simulink model "NLE_DiscreteSystem"  (R2024b)
settings: Solver=VariableStepAuto  StartTime=0.0  StopTime=20.0  RelTol=1e-3
values from neighbouring files (symbols this model uses):
  discrete_regulator = tf(Q, P, Ts)    [assignment1.m]
  disorder_times = [10, 14]    [assignment1.m]
  u_control = 0.5    [assignment1.m]
  z = 0.1    [assignment1.m]
settings Model: Creator=lukiq  LastModifiedBy=lukiq
settings DebuggingCC: AlgebraicLoopMsg=none

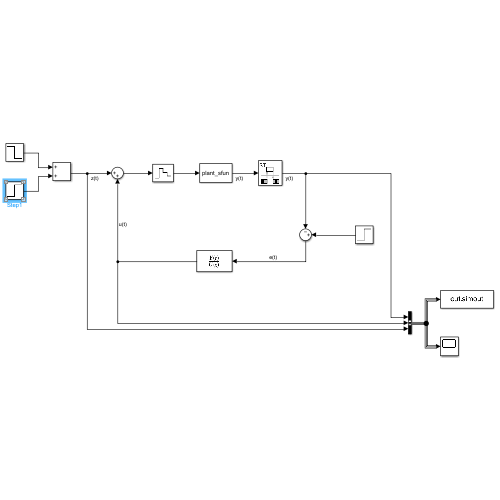
[thumbnail: Simulink's stored preview of the top-level diagram]
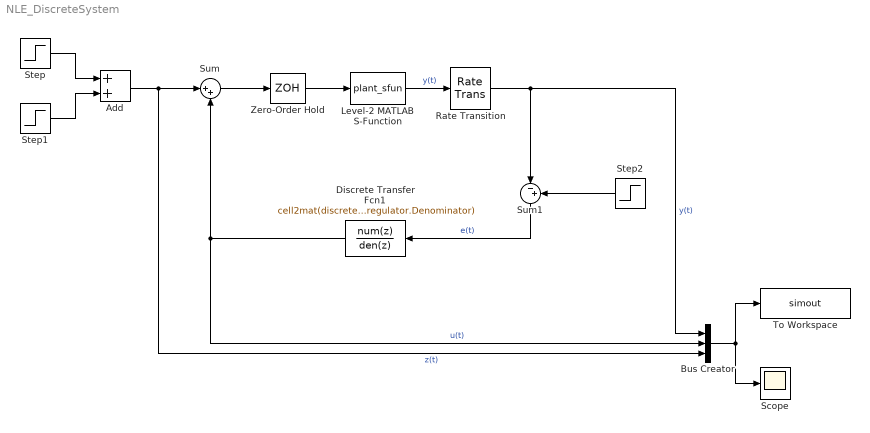
== system NLE_DiscreteSystem ==
  Add : Sum
  Bus Creator : BusCreator  Inputs=3
  Discrete Transfer Fcn1 : DiscreteTransferFcn  Numerator=cell2mat(discrete_regulator.Numerator)  Denominator=cell2mat(discrete_regulator.Denominator)
  Level-2 MATLAB S-Function : M-S-Function  FunctionName=plant_sfun  Parameters=odeHandleSimulink, p, u, outIdx
  Rate Transition : RateTransition
  Scope : Scope
  Step : Step  Time=disorder_times(1)  After=- z * u_control  SampleTime=0
  Step1 : Step  Time=disorder_times(2)  After=z * u_control  SampleTime=0
  Step2 : Step  Time=0  After=u_control  SampleTime=0
  Sum : Sum  Inputs=|++
  Sum1 : Sum  Inputs=|-+
  To Workspace : ToWorkspace  VariableName=simout  SaveFormat=Timeseries  SampleTime=-1
  Zero-Order Hold : ZeroOrderHold  SampleTime=-1
  wires:
  Discrete Transfer Fcn1/1 -> Bus Creator/2, Sum/2  "u(t)"
  Step/1 -> Add/1
  Add/1 -> Bus Creator/3, Sum/1  "z(t)"
  Step2/1 -> Sum1/2
  Sum1/1 -> Discrete Transfer Fcn1/1  "e(t)"
  Rate Transition/1 -> Bus Creator/1, Sum1/1  "y(t)"
  Step1/1 -> Add/2
  Bus Creator/1 -> Scope/1, To Workspace/1
  Zero-Order Hold/1 -> Level-2 MATLAB S-Function/1
  Sum/1 -> Zero-Order Hold/1
  Level-2 MATLAB S-Function/1 -> Rate Transition/1  "y(t)"
